simulink model "high"  (R2014a)
settings: Solver=FixedStepDiscrete  StartTime=0.0  StopTime=SimLength  FixedStep=0.01  RelTol=1e-3
undefined symbols (not defined in the file): SimLength
libraries: simulink x3
settings Model: Creator=Maik  LastModifiedBy=Jonas

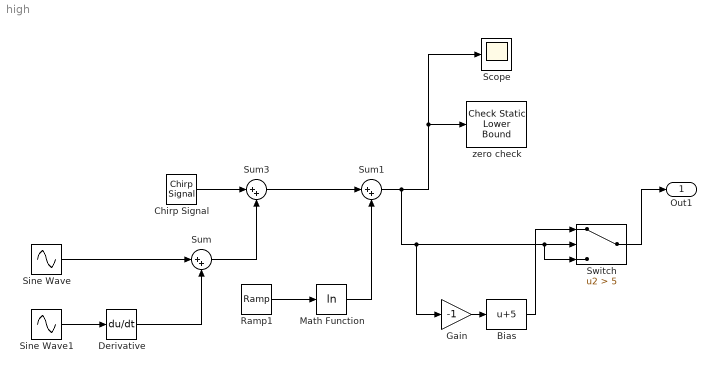
== system high ==
  Bias : Bias  Bias=5
  Chirp Signal : simulink/Sources/Chirp Signal  f1=0.2  T=SimLength  f2=0.7
  Derivative : Derivative
  Gain : Gain  Gain=-1
  Math Function : Math  Operator=log  SaturateOnIntegerOverflow=on
  Ramp1 : simulink/Sources/Ramp  slope=1  start=0  X0=1
  Scope : Scope
      settings: YMin=-1  YMax=1  SaveName=ScopeData5
  Sine Wave : Sin  Amplitude=0.2
  Sine Wave1 : Sin  Amplitude=0.2  Frequency=sqrt(3)
  Sum : Sum  Inputs=|++
  Sum1 : Sum  Inputs=|++
  Sum3 : Sum  Inputs=|++
  Switch : Switch  Criteria=u2 > Threshold  Threshold=5
  zero check : simulink/Model Verification/Check Static  Lower Bound  Description=0 <= u  min=0  min_included=on  enabled=on  stopWhenAssertionFail=on  export=off  icon=text
  Out1 : Outport
  wires:
  Sine Wave1/1 -> Derivative/1
  Sine Wave/1 -> Sum/1
  Derivative/1 -> Sum/2
  Sum1/1 -> Gain/1, Switch/3, Switch/2, Scope/1, zero check/1
  Ramp1/1 -> Math Function/1
  Math Function/1 -> Sum1/2
  Chirp Signal/1 -> Sum3/1
  Sum/1 -> Sum3/2
  Sum3/1 -> Sum1/1
  Gain/1 -> Bias/1
  Bias/1 -> Switch/1
  Switch/1 -> Out1/1
